simulink model "Plant_Model_W_Sensors_Un_biased"  (R2017b)
settings: Solver=VariableStepAuto  StartTime=0.0  StopTime=TF  FixedStep=0.001  MaxStep=1e-4  RelTol=1e-4
values from neighbouring files (symbols this model uses):
  Accel_bias = 1    [Model_W_MD_Sensors.m]
  Amps = C/1000    (= 0.7)    [Model_W_MD_Sensors.m]
  b = 1.144e-08    [Model_W_MD_Sensors.m]
  b_m = 2.415e-6    (= 2.415e-06)    [Model_W_MD_Sensors.m]
  CD = 0.7    [Model_W_MD_Sensors.m]
  d = 9.94e-10    [Model_W_MD_Sensors.m]
  g = 9.81    [Model_W_MD_Sensors.m]
  Grav_bias = g    (= 9.81)    [Model_W_MD_Sensors.m]
  Gyro_bias = .6    (= 0.6)    [Model_W_MD_Sensors.m]
  Ixx = 7.5*10^(-3)    (= 0.0075)    [Model_W_MD_Sensors.m]
  Iyy = 7.5*10^(-3)    (= 0.0075)    [Model_W_MD_Sensors.m]
  Izz = 1.3*10^(-2)    (= 0.013)    [Model_W_MD_Sensors.m]
  Jr = 6.5*10^(-7)    (= 6.5e-07)    [Model_W_MD_Sensors.m]
  Kemf = 0.00255    [Model_W_MD_Sensors.m]
  Kt = Kemf    (= 0.00255)    [Model_W_MD_Sensors.m]
  l = 0.23    [Model_W_MD_Sensors.m]
  L = 0.001*R    (= 0.000117)    [Model_W_MD_Sensors.m]
  m = weight/g    (= 0.0289500509684)    [Model_W_MD_Sensors.m]
  PD = 120    [Model_W_MD_Sensors.m]
  Phi_dot_bias = mean(Phi_dot)    [Model_W_MD_Sensors.m]
  Psi_dot_bias = mean(Psi_dot)    [Model_W_MD_Sensors.m]
  R = 0.117    [Model_W_MD_Sensors.m]
  Theta_dot_bias = mean(Theta_dot)    [Model_W_MD_Sensors.m]
  X_dot_dot_bias = mean(X_dot_dot)    [Model_W_MD_Sensors.m]
  Y_dot_dot_bias = mean(Y_dot_dot)    [Model_W_MD_Sensors.m]
  Z_dot_dot_bias = mean(Z_dot_dot)    [Model_W_MD_Sensors.m]
undefined symbols (not defined in the file or in its folder): Ion, Lithium
libraries: simulink x9, powerlib x2, electricdrivelib x1
settings Model: Creator=Nicky  LastModifiedBy=Nicky
settings SolverCC: ZeroCrossAlgorithm=Adaptive  AutoInsertRateTranBlk=on
settings DebuggingCC: MaxConsecutiveZCsMsg=none
settings CodeAppCC: StateflowObjectComments=on
settings SimscapeCC: SimscapeNormalizeSystem=off

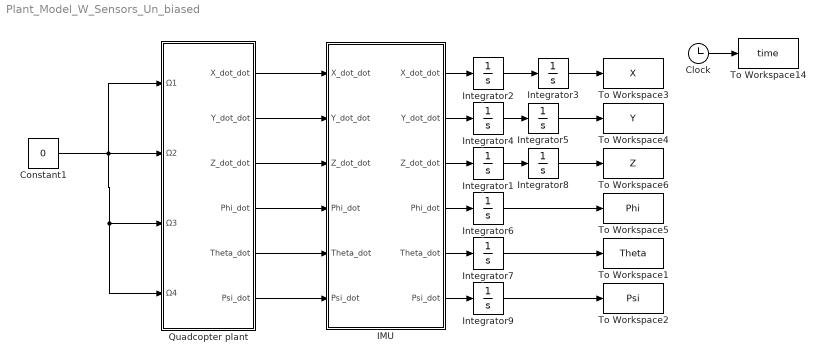
== system Plant_Model_W_Sensors_Un_biased ==
  Clock : Clock
  Constant1 : Constant  Value=0
  IMU : Subsystem
  Integrator{1..5,9} (6 alike) : Integrator
  Integrator6 : Integrator  WrapState=on
  Integrator7 : Integrator  WrapState=on
  Integrator8 : Integrator  LimitOutput=on  UpperSaturationLimit=0
  Quadcopter plant : Subsystem
  To Workspace1 : ToWorkspace  VariableName=Theta  SampleTime=0.001
      settings: Save2DSignal=2-D array (concatenate along first dimension)
  To Workspace14 : ToWorkspace  VariableName=time  SampleTime=0.001
      settings: Save2DSignal=2-D array (concatenate along first dimension)
  To Workspace2 : ToWorkspace  VariableName=Psi  SampleTime=0.001
      settings: Save2DSignal=2-D array (concatenate along first dimension)
  To Workspace3 : ToWorkspace  VariableName=X  SampleTime=0.001
      settings: Save2DSignal=2-D array (concatenate along first dimension)
  To Workspace4 : ToWorkspace  VariableName=Y  SampleTime=0.001
      settings: Save2DSignal=2-D array (concatenate along first dimension)
  To Workspace5 : ToWorkspace  VariableName=Phi  SampleTime=0.001
      settings: Save2DSignal=2-D array (concatenate along first dimension)
  To Workspace6 : ToWorkspace  VariableName=Z  SampleTime=0.001
      settings: Save2DSignal=2-D array (concatenate along first dimension)
  wires:
  Clock/1 -> To Workspace14/1
  Quadcopter plant/1(X_dot_dot) -> IMU/1(X_dot_dot)
  Quadcopter plant/2("Y_dot_dot ") -> IMU/2(Y_dot_dot)
  Quadcopter plant/3(Z_dot_dot) -> IMU/3(Z_dot_dot)
  Quadcopter plant/4(Phi_dot) -> IMU/4(Phi_dot)
  Quadcopter plant/5(Theta_dot) -> IMU/5(Theta_dot)
  Quadcopter plant/6(Psi_dot) -> IMU/6(Psi_dot)
  Constant1/1 -> Quadcopter plant/1(Ω1), Quadcopter plant/2(Ω2), Quadcopter plant/3(Ω3), Quadcopter plant/4(Ω4)
  Integrator4/1 -> Integrator5/1
  Integrator2/1 -> Integrator3/1
  Integrator3/1 -> To Workspace3/1
  IMU/1("X_dot_dot ") -> Integrator2/1
  IMU/2("Y_dot_dot ") -> Integrator4/1
  Integrator5/1 -> To Workspace4/1
  Integrator1/1 -> Integrator8/1
  IMU/3("Z_dot_dot ") -> Integrator1/1
  Integrator8/1 -> To Workspace6/1
  IMU/4("Phi_dot ") -> Integrator6/1
  Integrator6/1 -> To Workspace5/1
  IMU/5("Theta_dot ") -> Integrator7/1
  Integrator7/1 -> To Workspace1/1
  IMU/6("Psi_dot ") -> Integrator9/1
  Integrator9/1 -> To Workspace2/1

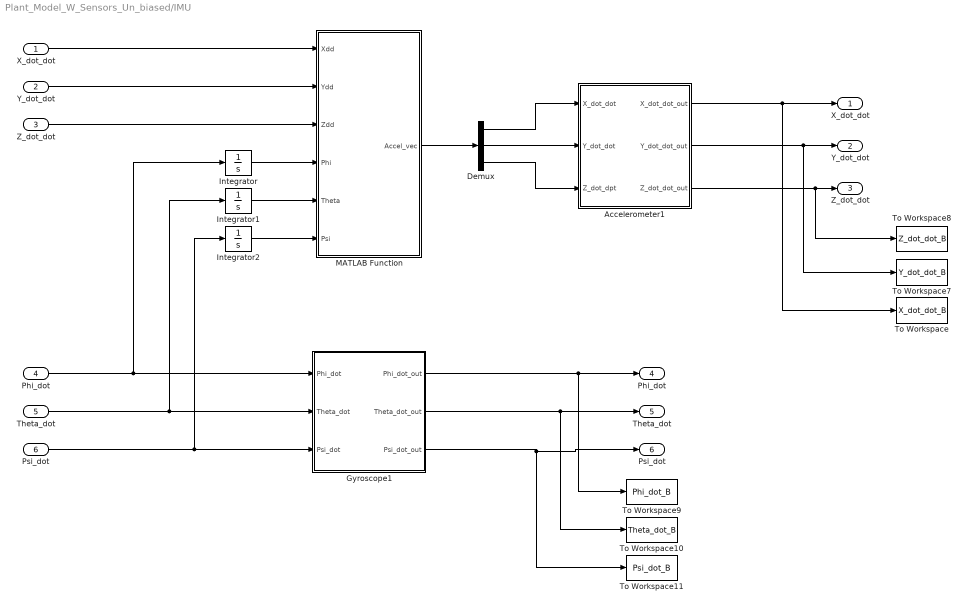
== system Plant_Model_W_Sensors_Un_biased/IMU ==
  X_dot_dot : Inport
  Y_dot_dot : Inport  Port=2
  Z_dot_dot : Inport  Port=3
  Phi_dot : Inport  Port=4
  Theta_dot : Inport  Port=5
  Psi_dot : Inport  Port=6
  Accelerometer1 : Subsystem
  Demux : Demux  Outputs=3
  Gyroscope1 : Subsystem
  Integrator : Integrator  WrapState=on
  Integrator1 : Integrator  WrapState=on
  Integrator2 : Integrator
  MATLAB Function : MATLAB Function  TreatAsAtomicUnit=on
  To Workspace : ToWorkspace  VariableName=X_dot_dot_B  SampleTime=0.001
      settings: Save2DSignal=2-D array (concatenate along first dimension)
  To Workspace10 : ToWorkspace  VariableName=Theta_dot_B  SampleTime=0.001
      settings: Save2DSignal=2-D array (concatenate along first dimension)
  To Workspace11 : ToWorkspace  VariableName=Psi_dot_B  SampleTime=0.001
      settings: Save2DSignal=2-D array (concatenate along first dimension)
  To Workspace7 : ToWorkspace  VariableName=Y_dot_dot_B  SampleTime=0.001
      settings: Save2DSignal=2-D array (concatenate along first dimension)
  To Workspace8 : ToWorkspace  VariableName=Z_dot_dot_B  SampleTime=0.001
      settings: Save2DSignal=2-D array (concatenate along first dimension)
  To Workspace9 : ToWorkspace  VariableName=Phi_dot_B  SampleTime=0.001
      settings: Save2DSignal=2-D array (concatenate along first dimension)
  "X_dot_dot " : Outport
  "Y_dot_dot " : Outport  Port=2
  "Z_dot_dot " : Outport  Port=3
  "Phi_dot " : Outport  Port=4
  "Theta_dot " : Outport  Port=5
  "Psi_dot " : Outport  Port=6
  wires:
  Phi_dot/1 -> Gyroscope1/1(Phi_dot), Integrator/1
  Theta_dot/1 -> Gyroscope1/2(Theta_dot), Integrator1/1
  Psi_dot/1 -> Gyroscope1/3(Psi_dot), Integrator2/1
  X_dot_dot/1 -> MATLAB Function/1(Xdd)
  Y_dot_dot/1 -> MATLAB Function/2(Ydd)
  Z_dot_dot/1 -> MATLAB Function/3(Zdd)
  Integrator/1 -> MATLAB Function/4(Phi)
  Integrator2/1 -> MATLAB Function/6(Psi)
  Integrator1/1 -> MATLAB Function/5(Theta)
  MATLAB Function/1(Accel_vec) -> Demux/1
  Demux/2 -> Accelerometer1/2("Y_dot_dot ")
  Demux/1 -> Accelerometer1/1(X_dot_dot)
  Demux/3 -> Accelerometer1/3("Z_dot_dpt ")
  Accelerometer1/2(Y_dot_dot_out) -> To Workspace7/1, "Y_dot_dot "/1
  Accelerometer1/3(Z_dot_dot_out) -> "Z_dot_dot "/1, To Workspace8/1
  Accelerometer1/1(X_dot_dot_out) -> "X_dot_dot "/1, To Workspace/1
  Gyroscope1/2(Theta_dot_out) -> "Theta_dot "/1, To Workspace10/1
  Gyroscope1/1(Phi_dot_out) -> "Phi_dot "/1, To Workspace9/1
  Gyroscope1/3(Psi_dot_out) -> "Psi_dot "/1, To Workspace11/1

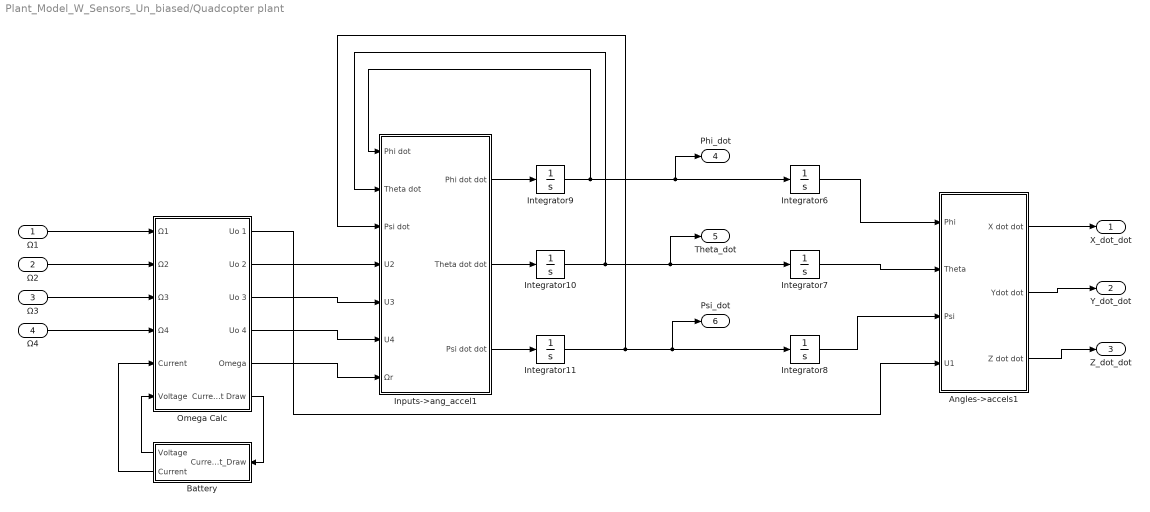
== system Plant_Model_W_Sensors_Un_biased/Quadcopter plant ==
  Ω1 : Inport
  Ω2 : Inport  Port=2
  Ω3 : Inport  Port=3
  Ω4 : Inport  Port=4
  Angles->accels1 : Subsystem
  Battery : Subsystem
  Inputs->ang_accel1 : Subsystem
  Integrator10 : Integrator  IgnoreLimit=on
  Integrator11 : Integrator  UpperSaturationLimit=10000  LowerSaturationLimit=-10000
  Integrator6 : Integrator  WrapState=on
  Integrator7 : Integrator  WrapState=on
  Integrator8 : Integrator
  Integrator9 : Integrator
  Omega Calc : Subsystem
  X_dot_dot : Outport
  "Y_dot_dot " : Outport  Port=2
  Z_dot_dot : Outport  Port=3
  Phi_dot : Outport  Port=4
  Theta_dot : Outport  Port=5
  Psi_dot : Outport  Port=6
  wires:
  Integrator8/1 -> Angles->accels1/3(Psi)
  Integrator7/1 -> Angles->accels1/2(Theta)
  Integrator6/1 -> Angles->accels1/1(Phi)
  Inputs->ang_accel1/2(Theta dot dot) -> Integrator10/1
  Inputs->ang_accel1/1(Phi dot dot) -> Integrator9/1
  Inputs->ang_accel1/3(Psi dot dot) -> Integrator11/1
  Omega Calc/5(Omega) -> Inputs->ang_accel1/7(Ωr)
  Omega Calc/4(Uo 4) -> Inputs->ang_accel1/6(U4)
  Omega Calc/3(Uo 3) -> Inputs->ang_accel1/5(U3)
  Omega Calc/2(Uo 2) -> Inputs->ang_accel1/4(U2)
  Omega Calc/1(Uo 1) -> Angles->accels1/4(U1)
  Ω1/1 -> Omega Calc/1(Ω1)
  Ω2/1 -> Omega Calc/2(Ω2)
  Ω3/1 -> Omega Calc/3(Ω3)
  Ω4/1 -> Omega Calc/4(Ω4)
  Integrator9/1 -> Inputs->ang_accel1/1(Phi dot), Phi_dot/1, Integrator6/1
  Integrator11/1 -> Inputs->ang_accel1/3(Psi dot), Integrator8/1, Psi_dot/1
  Integrator10/1 -> Inputs->ang_accel1/2(Theta dot), Integrator7/1, Theta_dot/1
  Angles->accels1/1(X dot dot) -> X_dot_dot/1
  Angles->accels1/2(Ydot dot) -> "Y_dot_dot "/1
  Angles->accels1/3(Z dot dot) -> Z_dot_dot/1
  Omega Calc/6(Current Draw) -> Battery/1(Current_Draw)
  Battery/1(Voltage) -> Omega Calc/6(Voltage)
  Battery/2(Current) -> Omega Calc/5(Current)

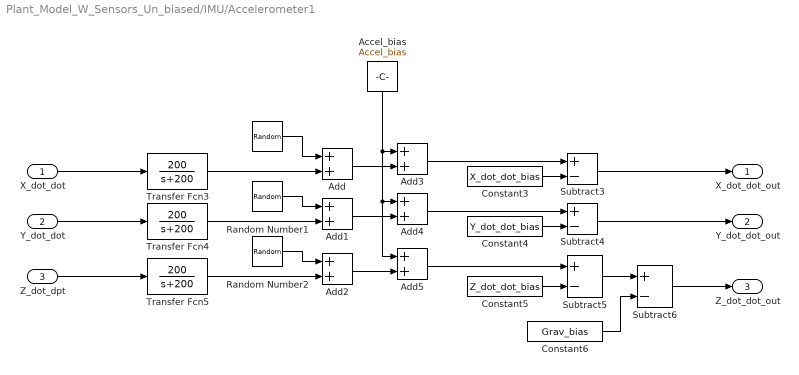
== system Plant_Model_W_Sensors_Un_biased/IMU/Accelerometer1 ==
  X_dot_dot : Inport
  "Y_dot_dot " : Inport  Port=2
  "Z_dot_dpt " : Inport  Port=3
  " " : RandomNumber  Variance=0.0001  Seed=1  SampleTime=0.001
  Accel_bias : Constant  Value=Accel_bias
  Add{,1..5} (6 alike) : Sum
  Constant3 : Constant  Value=X_dot_dot_bias
  Constant4 : Constant  Value=Y_dot_dot_bias
  Constant5 : Constant  Value=Z_dot_dot_bias
  Constant6 : Constant  Value=Grav_bias
  Random Number1 : RandomNumber  Variance=0.0001  Seed=2  SampleTime=0.001
  Random Number2 : RandomNumber  Mean=0.000  Variance=0.0001  Seed=3  SampleTime=0.001
  Subtract{3..6} (4 alike) : Sum  Inputs=+-
  Transfer Fcn3 : TransferFcn  Numerator=[200]  Denominator=[1 200]
  Transfer Fcn4 : TransferFcn  Numerator=[200]  Denominator=[1 200]
  Transfer Fcn5 : TransferFcn  Numerator=[200]  Denominator=[1 200]
  X_dot_dot_out : Outport
  Y_dot_dot_out : Outport  Port=2
  Z_dot_dot_out : Outport  Port=3
  wires:
  Constant6/1 -> Subtract6/2
  Constant4/1 -> Subtract4/2
  Constant3/1 -> Subtract3/2
  Constant5/1 -> Subtract5/2
  Subtract5/1 -> Subtract6/1
  X_dot_dot/1 -> Transfer Fcn3/1
  "Y_dot_dot "/1 -> Transfer Fcn4/1
  Accel_bias/1 -> Add5/1, Add4/1, Add3/1
  Add/1 -> Add3/2
  Add2/1 -> Add5/2
  Add1/1 -> Add4/2
  Add3/1 -> Subtract3/1
  Add4/1 -> Subtract4/1
  Add5/1 -> Subtract5/1
  " "/1 -> Add/1
  Random Number1/1 -> Add1/1
  Random Number2/1 -> Add2/1
  "Z_dot_dpt "/1 -> Transfer Fcn5/1
  Subtract3/1 -> X_dot_dot_out/1
  Subtract4/1 -> Y_dot_dot_out/1
  Subtract6/1 -> Z_dot_dot_out/1
  Transfer Fcn3/1 -> Add/2
  Transfer Fcn5/1 -> Add2/2
  Transfer Fcn4/1 -> Add1/2

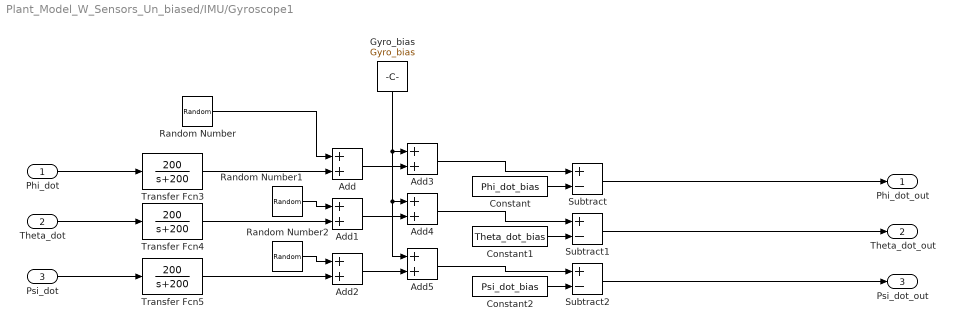
== system Plant_Model_W_Sensors_Un_biased/IMU/Gyroscope1 ==
  Phi_dot : Inport
  Theta_dot : Inport  Port=2
  Psi_dot : Inport  Port=3
  Add{,1..5} (6 alike) : Sum
  Constant : Constant  Value=Phi_dot_bias
  Constant1 : Constant  Value=Theta_dot_bias
  Constant2 : Constant  Value=Psi_dot_bias
  Gyro_bias : Constant  Value=Gyro_bias
  Random Number : RandomNumber  Variance=0.0001  Seed=4  SampleTime=0.001
  Random Number1 : RandomNumber  Variance=0.0001  Seed=5  SampleTime=0.001
  Random Number2 : RandomNumber  Variance=0.0001  Seed=6  SampleTime=0.001
  Subtract : Sum  Inputs=+-
  Subtract1 : Sum  Inputs=+-
  Subtract2 : Sum  Inputs=+-
  Transfer Fcn3 : TransferFcn  Numerator=[200]  Denominator=[1 200]
  Transfer Fcn4 : TransferFcn  Numerator=[200]  Denominator=[1 200]
  Transfer Fcn5 : TransferFcn  Numerator=[200]  Denominator=[1 200]
  Phi_dot_out : Outport
  Theta_dot_out : Outport  Port=2
  Psi_dot_out : Outport  Port=3
  wires:
  Constant/1 -> Subtract/2
  Constant2/1 -> Subtract2/2
  Constant1/1 -> Subtract1/2
  Phi_dot/1 -> Transfer Fcn3/1
  Theta_dot/1 -> Transfer Fcn4/1
  Psi_dot/1 -> Transfer Fcn5/1
  Add/1 -> Add3/2
  Add1/1 -> Add4/2
  Add2/1 -> Add5/2
  Add5/1 -> Subtract2/1
  Add3/1 -> Subtract/1
  Add4/1 -> Subtract1/1
  Gyro_bias/1 -> Add5/1, Add4/1, Add3/1
  Random Number/1 -> Add/1
  Random Number1/1 -> Add1/1
  Random Number2/1 -> Add2/1
  Subtract/1 -> Phi_dot_out/1
  Subtract1/1 -> Theta_dot_out/1
  Subtract2/1 -> Psi_dot_out/1
  Transfer Fcn3/1 -> Add/2
  Transfer Fcn5/1 -> Add2/2
  Transfer Fcn4/1 -> Add1/2

== system Plant_Model_W_Sensors_Un_biased/Quadcopter plant/Angles->accels1 ==
  Phi : Inport
  Theta : Inport  Port=2
  Psi : Inport  Port=3
  U1 : Inport  Port=4
  Constant : Constant  Value=m
  Divide : Product  Inputs=*/
  Subsystem : Subsystem
  Subsystem1 : Subsystem
  Subsystem2 : Subsystem
  X dot dot : Outport
  Ydot dot : Outport  Port=2
  Z dot dot : Outport  Port=3
  wires:
  Phi/1 -> Subsystem1/1(Phi), Subsystem2/1(Phi), Subsystem/1(Phi)
  U1/1 -> Divide/1
  Constant/1 -> Divide/2
  Divide/1 -> Subsystem2/3(U1/m), Subsystem1/4(U1/M), Subsystem/4(U1/M)
  Subsystem/1(X_dot_dot) -> X dot dot/1
  Subsystem1/1(Y_dot_dot) -> Ydot dot/1
  Subsystem2/1(Z_dot_dot) -> Z dot dot/1
  Theta/1 -> Subsystem2/2(Theta), Subsystem1/2(Theta), Subsystem/2(Theta)
  Psi/1 -> Subsystem/3(Psi), Subsystem1/3(Psi)

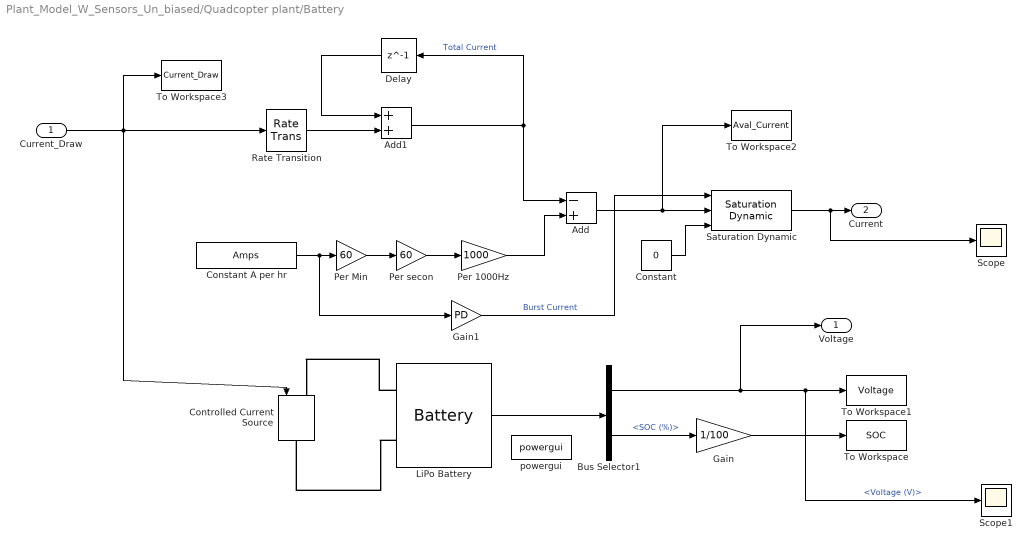
== system Plant_Model_W_Sensors_Un_biased/Quadcopter plant/Battery ==
  Current_Draw : Inport
  Add : Sum  Inputs=-+
  Add1 : Sum
  Bus Selector1 : BusSelector  OutputSignals=Voltage (V),SOC (%)
  Constant : Constant  Value=0
  Constant A per hr : Constant  Value=Amps
  Controlled Current Source : powerlib/Electrical Sources/Controlled Current Source  Initialize=on  Source_Type=DC  Amplitude=0  Phase=0  Frequency=0  Measurements=None
  Delay : Delay  DelayLength=1  InitialCondition=0
  Gain : Gain  Gain=1/100
  Gain1 : Gain  Gain=PD
  "LiPo Battery " : electricdrivelib/Extra Sources/Battery  BatType=Lithium-Ion  ShowTempParam=off  ThermalPreset=no  ShowAgeParam=off  NomV=11.1  NomQ=.7  SOC=100  Batt_Tr=1  PresetModel=off  MaxQ=0.7  MinV=8.325  FullV=11.75  Dis_rate=.7  R=.08  Normal_OP=.7  expZone="[11.75   0.5]"  current=CD*Amps  Units=Ampere-hour  Tci=20  NomT=25  T2=0  MaxQ2=2.208  FullV2=3.45  Normal_OP2=2.8  expZone2="[3.22        0.23]"  Rca=0.6  ti=1000  Dp=0  Neq0=0  Tsim=1e6  Ta1=25  Qeol=5.4*0.9  Reol=0.013333*1.2  Char_age=[2.3478, 3]  Dis_age=[2.3478, 10]  N1=1500  N2=10500  N3=1000  N4=1400  Ta2=45  N5=950
  Per 1000Hz : Gain  Gain=1000
  Per Min : Gain  Gain=60
  Per secon : Gain  Gain=60
  Rate Transition : RateTransition  OutPortSampleTimeMultiple=0  OutPortSampleTime=0.001
  Saturation Dynamic : simulink/Discontinuities/Saturation Dynamic  OutMin=[]  OutMax=[]  OutDataTypeStr=Inherit: Same as second input  OutDataType=fixdt(1, 16)  OutScaling=2^-10  DoSatur=off
  Scope : Scope
  Scope1 : Scope
  To Workspace : ToWorkspace  VariableName=SOC  SampleTime=.1
      settings: Save2DSignal=2-D array (concatenate along first dimension)
  To Workspace1 : ToWorkspace  VariableName=Voltage  SampleTime=.1
      settings: Save2DSignal=2-D array (concatenate along first dimension)
  To Workspace2 : ToWorkspace  VariableName=Aval_Current  SampleTime=.1
      settings: Save2DSignal=2-D array (concatenate along first dimension)
  To Workspace3 : ToWorkspace  VariableName=Current_Draw  SampleTime=.1
      settings: Save2DSignal=2-D array (concatenate along first dimension)
  powergui : powerlib/powergui  SimulationMode=Continuous  SampleTime=0.001  frequency=60  Iterations=50  frequencyindice=0  Pbase=100e6  ErrMax=1e-4  UnitsV=kV  UnitsW=MW  buscounter=0  FunctionMessages=off  echomessages=off  EnableUseOfTLC=off  CurrentSourceSwitches=off  DisableSnubberDevices=off  DisableRonSwitches=off  DisableVfSwitches=off  DisplayEquations=off  SolverType=Tustin/Backward Euler (TBE)  Interpol=off  ExternalGateDelay=off  methode=off  Ts=100  x0status=blocks  SPID=on  SwTol=0  HookPort=off  RestoreLinks=warning  ResistiveCurrentMeasurement=off  Frange=[0:2:500]  Ylog=off  Xlog=on  ShowGrid=off  save=off  variable=ZData  structure=0  ZoomFFT=on  StartTime=0.0  cycles=1  DisplayStyle=1  fundamental=60  FreqAxis=off  MaxFrequency=1000  frequencyindicesteady=1  RmsSteady=1  display=off
  Voltage : Outport
  Current : Outport  Port=2
  wires:
  Per Min/1 -> Per secon/1
  Constant A per hr/1 -> Gain1/1, Per Min/1
  Per secon/1 -> Per 1000Hz/1
  Per 1000Hz/1 -> Add/2
  Add1/1 -> Add/1, Delay/1  "Total Current"
  Rate Transition/1 -> Add1/2
  Delay/1 -> Add1/1
  Constant/1 -> Saturation Dynamic/3
  Current_Draw/1 -> To Workspace3/1, Controlled Current Source/1, Rate Transition/1
  Bus Selector1/1 -> Voltage/1, Scope1/1, To Workspace1/1  "<Voltage (V)>"
  Bus Selector1/2 -> Gain/1  "<SOC (%)>"
  Gain/1 -> To Workspace/1
  "LiPo Battery "/1 -> Bus Selector1/1
  Add/1 -> To Workspace2/1, Saturation Dynamic/2
  Saturation Dynamic/1 -> Scope/1, Current/1
  Gain1/1 -> Saturation Dynamic/1  "Burst Current"
  connections:
  "LiPo Battery "/LConn1 -- Controlled Current Source/LConn1
  "LiPo Battery "/LConn2 -- Controlled Current Source/RConn1

== system Plant_Model_W_Sensors_Un_biased/Quadcopter plant/Inputs->ang_accel1 ==
  Phi dot : Inport
  Theta dot : Inport  Port=2
  Psi dot : Inport  Port=3
  U2 : Inport  Port=4
  U3 : Inport  Port=5
  U4 : Inport  Port=6
  Ωr : Inport  Port=7
  Subsystem : Subsystem
  Subsystem1 : Subsystem
  Subsystem2 : Subsystem
  Phi dot dot : Outport
  Theta dot dot : Outport  Port=2
  Psi dot dot : Outport  Port=3
  wires:
  U3/1 -> Subsystem2/3(U3)
  U4/1 -> Subsystem1/3(U4)
  Subsystem/1(Phi_dot_dot) -> Phi dot dot/1
  U2/1 -> Subsystem/1(U2)
  Ωr/1 -> Subsystem/4(Ωr), Subsystem2/1(Ωr)
  Psi dot/1 -> Subsystem2/2(Psi_dot), Subsystem/3(Psi_dot)
  Subsystem2/1(Theta_dot_dot) -> Theta dot dot/1
  Subsystem1/1(Psi_dot_dot) -> Psi dot dot/1
  Theta dot/1 -> Subsystem/2(Theta_dot), Subsystem1/2(Theta_dot)
  Phi dot/1 -> Subsystem2/4(Phi_dot), Subsystem1/1(Phi_dot)

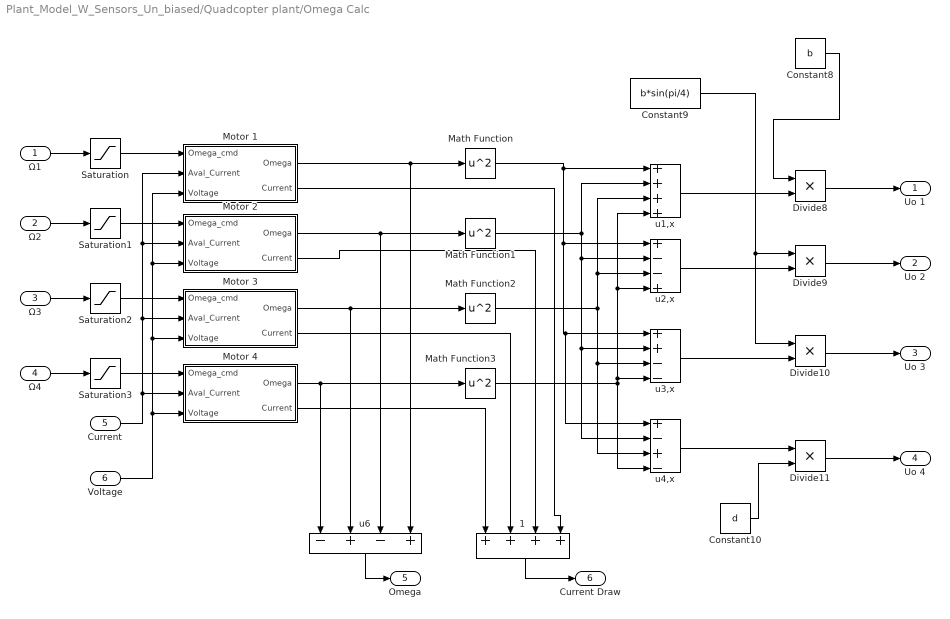
== system Plant_Model_W_Sensors_Un_biased/Quadcopter plant/Omega Calc ==
  Ω1 : Inport
  Ω2 : Inport  Port=2
  Ω3 : Inport  Port=3
  Ω4 : Inport  Port=4
  Current : Inport  Port=5
  Voltage : Inport  Port=6
  " 1" : Sum  Inputs=++++
  " Motor 1" : Subsystem
  " Motor 2" : Subsystem
  " Motor 3" : Subsystem
  " Motor 4" : Subsystem
  Constant10 : Constant  Value=d
  Constant8 : Constant  Value=b
  Constant9 : Constant  Value=b*sin(pi/4)
  Divide{8..11} (4 alike) : Product  Inputs=**
  Math Function{,1..3} (4 alike) : Math  Operator=square  SaturateOnIntegerOverflow=on
  Saturation{,1..3} (4 alike) : Saturate  UpperLimit=inf  LowerLimit=0
  u1,x : Sum  Inputs=++++
  u2,x : Sum  Inputs=+--+
  u3,x : Sum  Inputs=++--
  u4,x : Sum  Inputs=+-+-
  u6 : Sum  Inputs=-+-+
  Uo 1 : Outport
  Uo 2 : Outport  Port=2
  Uo 3 : Outport  Port=3
  Uo 4 : Outport  Port=4
  Omega : Outport  Port=5
  Current Draw : Outport  Port=6
  wires:
  Constant10/1 -> Divide11/2
  u4,x/1 -> Divide11/1
  u3,x/1 -> Divide10/2
  u2,x/1 -> Divide9/2
  Constant9/1 -> Divide10/1, Divide9/1
  u1,x/1 -> Divide8/2
  Constant8/1 -> Divide8/1
  u6/1 -> Omega/1
  Divide8/1 -> Uo 1/1
  Divide9/1 -> Uo 2/1
  Divide10/1 -> Uo 3/1
  Divide11/1 -> Uo 4/1
  " Motor 1"/1(Omega) -> u6/4, Math Function/1
  " Motor 2"/1(Omega) -> u6/3, Math Function1/1
  " Motor 3"/1(Omega) -> u6/2, Math Function2/1
  " Motor 4"/1(Omega) -> u6/1, Math Function3/1
  " 1"/1 -> Current Draw/1
  Ω1/1 -> Saturation/1
  Ω2/1 -> Saturation1/1
  Ω3/1 -> Saturation2/1
  Ω4/1 -> Saturation3/1
  Saturation/1 -> " Motor 1"/1(Omega_cmd)
  Saturation1/1 -> " Motor 2"/1(Omega_cmd)
  Saturation2/1 -> " Motor 3"/1(Omega_cmd)
  Saturation3/1 -> " Motor 4"/1(Omega_cmd)
  Current/1 -> " Motor 4"/2(Aval_Current), " Motor 3"/2(Aval_Current), " Motor 2"/2(Aval_Current), " Motor 1"/2(Aval_Current)
  Voltage/1 -> " Motor 4"/3(Voltage), " Motor 3"/3(Voltage), " Motor 2"/3(Voltage), " Motor 1"/3(Voltage)
  " Motor 4"/2("Current ") -> " 1"/1
  " Motor 3"/2("Current ") -> " 1"/2
  " Motor 2"/2("Current ") -> " 1"/3
  " Motor 1"/2("Current ") -> " 1"/4
  Math Function/1 -> u4,x/1, u3,x/1, u2,x/1, u1,x/1
  Math Function1/1 -> u4,x/2, u3,x/2, u2,x/2, u1,x/2
  Math Function2/1 -> u4,x/3, u3,x/3, u1,x/3, u2,x/3
  Math Function3/1 -> u4,x/4, u1,x/4, u2,x/4, u3,x/4

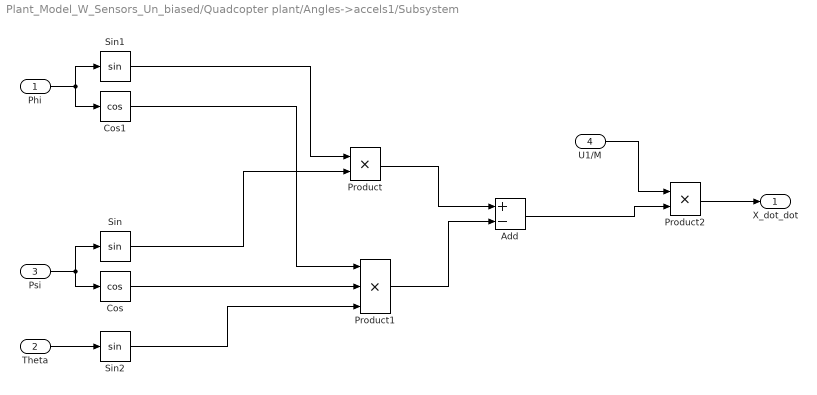
== system Plant_Model_W_Sensors_Un_biased/Quadcopter plant/Angles->accels1/Subsystem ==
  Phi : Inport
  Theta : Inport  Port=2
  Psi : Inport  Port=3
  U1/M : Inport  Port=4
  Add : Sum  Inputs=+-
  Cos : Trigonometry  Operator=cos
  Cos1 : Trigonometry  Operator=cos
  Product : Product
  Product1 : Product  Inputs=3
  Product2 : Product
  Sin : Trigonometry
  Sin1 : Trigonometry
  Sin2 : Trigonometry
  X_dot_dot : Outport
  wires:
  Product2/1 -> X_dot_dot/1
  Product1/1 -> Add/2
  Product/1 -> Add/1
  U1/M/1 -> Product2/1
  Add/1 -> Product2/2
  Psi/1 -> Cos/1, Sin/1
  Phi/1 -> Cos1/1, Sin1/1
  Theta/1 -> Sin2/1
  Cos1/1 -> Product1/1
  Cos/1 -> Product1/2
  Sin2/1 -> Product1/3
  Sin1/1 -> Product/1
  Sin/1 -> Product/2

== system Plant_Model_W_Sensors_Un_biased/Quadcopter plant/Angles->accels1/Subsystem1 ==
  Phi : Inport
  Theta : Inport  Port=2
  Psi : Inport  Port=3
  U1/M : Inport  Port=4
  Add1 : Sum
  Cos : Trigonometry  Operator=cos
  Cos1 : Trigonometry  Operator=cos
  Product3 : Product
  Product4 : Product  Inputs=3
  Product5 : Product
  Sin : Trigonometry
  Sin1 : Trigonometry
  Sin2 : Trigonometry
  Y_dot_dot : Outport
  wires:
  Psi/1 -> Sin/1, Cos/1
  Phi/1 -> Cos1/1, Sin1/1
  Theta/1 -> Sin2/1
  Product5/1 -> Y_dot_dot/1
  Add1/1 -> Product5/2
  Product4/1 -> Add1/2
  U1/M/1 -> Product5/1
  Product3/1 -> Add1/1
  Cos1/1 -> Product4/1
  Sin/1 -> Product4/2
  Sin2/1 -> Product4/3
  Sin1/1 -> Product3/1
  Cos/1 -> Product3/2

== system Plant_Model_W_Sensors_Un_biased/Quadcopter plant/Angles->accels1/Subsystem2 ==
  Phi : Inport
  Theta : Inport  Port=2
  U1/m : Inport  Port=3
  Add2 : Sum  Inputs=+-
  Constant2 : Constant  Value=g
  Cos : Trigonometry  Operator=cos
  Cos1 : Trigonometry  Operator=cos
  Product6 : Product  Inputs=3
  Z_dot_dot : Outport
  wires:
  Phi/1 -> Cos1/1
  Theta/1 -> Cos/1
  U1/m/1 -> Product6/3
  Constant2/1 -> Add2/1
  Cos/1 -> Product6/1
  Product6/1 -> Add2/2
  Cos1/1 -> Product6/2
  Add2/1 -> Z_dot_dot/1

== system Plant_Model_W_Sensors_Un_biased/Quadcopter plant/Inputs->ang_accel1/Subsystem ==
  U2 : Inport
  Theta_dot : Inport  Port=2
  Psi_dot : Inport  Port=3
  Ωr : Inport  Port=4
  Add : Sum  Inputs=+++
  Constant : Constant  Value=Iyy-Izz
  Constant1 : Constant  Value=Jr
  Constant2 : Constant  Value=l
  Constant3 : Constant  Value=Ixx
  Divide : Product  Inputs=*/
  Product : Product  Inputs=3
  Product1 : Product  Inputs=3
  Product2 : Product
  Phi_dot_dot : Outport
  wires:
  Psi_dot/1 -> Product/2
  Theta_dot/1 -> Product/1, Product1/3
  Constant/1 -> Product/3
  Ωr/1 -> Product1/2
  Constant1/1 -> Product1/1
  U2/1 -> Product2/2
  Constant2/1 -> Product2/1
  Product1/1 -> Add/2
  Product2/1 -> Add/1
  Product/1 -> Add/3
  Add/1 -> Divide/1
  Constant3/1 -> Divide/2
  Divide/1 -> Phi_dot_dot/1

== system Plant_Model_W_Sensors_Un_biased/Quadcopter plant/Inputs->ang_accel1/Subsystem1 ==
  Phi_dot : Inport
  Theta_dot : Inport  Port=2
  U4 : Inport  Port=3
  Add2 : Sum
  Constant11 : Constant  Value=Izz
  Constant8 : Constant  Value=Ixx-Iyy
  Divide2 : Product  Inputs=*/
  Product6 : Product  Inputs=3
  Psi_dot_dot : Outport
  wires:
  Theta_dot/1 -> Product6/1
  Phi_dot/1 -> Product6/2
  Constant8/1 -> Product6/3
  Add2/1 -> Divide2/1
  Constant11/1 -> Divide2/2
  Divide2/1 -> Psi_dot_dot/1
  Product6/1 -> Add2/2
  U4/1 -> Add2/1

== system Plant_Model_W_Sensors_Un_biased/Quadcopter plant/Inputs->ang_accel1/Subsystem2 ==
  Ωr : Inport
  Psi_dot : Inport  Port=2
  U3 : Inport  Port=3
  Phi_dot : Inport  Port=4
  Add1 : Sum  Inputs=+-+
  Constant4 : Constant  Value=Izz-Ixx
  Constant5 : Constant  Value=Jr
  Constant6 : Constant  Value=l
  Constant7 : Constant  Value=Iyy
  Divide1 : Product  Inputs=*/
  Product3 : Product  Inputs=3
  Product4 : Product  Inputs=3
  Product5 : Product
  Theta_dot_dot : Outport
  wires:
  Psi_dot/1 -> Product3/2
  Phi_dot/1 -> Product3/1, Product4/3
  Ωr/1 -> Product4/2
  Constant4/1 -> Product3/3
  Constant5/1 -> Product4/1
  U3/1 -> Product5/2
  Constant6/1 -> Product5/1
  Product4/1 -> Add1/2
  Product5/1 -> Add1/1
  Product3/1 -> Add1/3
  Add1/1 -> Divide1/1
  Constant7/1 -> Divide1/2
  Divide1/1 -> Theta_dot_dot/1

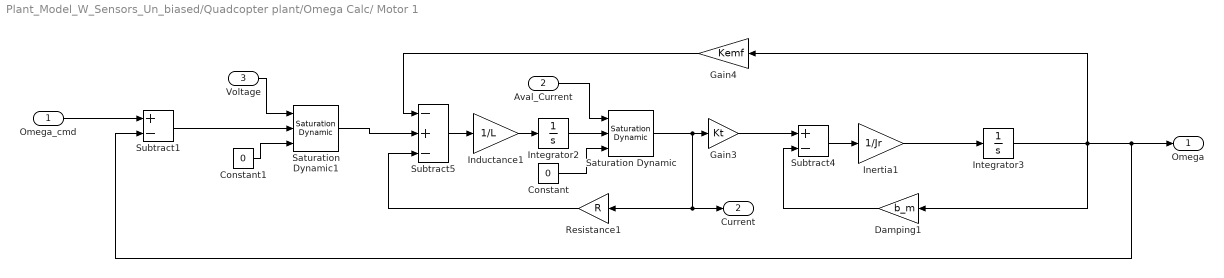
== system Plant_Model_W_Sensors_Un_biased/Quadcopter plant/Omega Calc/ Motor 1 ==
  Omega_cmd : Inport
  Aval_Current : Inport  Port=2
  Voltage : Inport  Port=3
  Constant : Constant  Value=0
  Constant1 : Constant  Value=0
  Damping1 : Gain  Gain=b_m
  Gain3 : Gain  Gain=Kt
  Gain4 : Gain  Gain=Kemf
  Inductance1 : Gain  Gain=1/L
  Inertia1 : Gain  Gain=1/Jr
  Integrator2 : Integrator  LimitOutput=on  LowerSaturationLimit=0
  Integrator3 : Integrator  LimitOutput=on  LowerSaturationLimit=0
  Resistance1 : Gain  Gain=R
  Saturation Dynamic : simulink/Discontinuities/Saturation Dynamic  OutMin=[]  OutMax=[]  OutDataTypeStr=Inherit: Same as second input  OutDataType=fixdt(1, 16)  OutScaling=2^-10  DoSatur=off
  Saturation Dynamic1 : simulink/Discontinuities/Saturation Dynamic  OutMin=[]  OutMax=[]  OutDataTypeStr=Inherit: Same as second input  OutDataType=fixdt(1, 16)  OutScaling=2^-10  DoSatur=off
  Subtract1 : Sum  Inputs=+-
  Subtract4 : Sum  Inputs=+-
  Subtract5 : Sum  Inputs=-+-
  Omega : Outport
  "Current " : Outport  Port=2
  wires:
  Inductance1/1 -> Integrator2/1
  Inertia1/1 -> Integrator3/1
  Resistance1/1 -> Subtract5/3
  Damping1/1 -> Subtract4/2
  Subtract5/1 -> Inductance1/1
  Saturation Dynamic1/1 -> Subtract5/2
  Gain4/1 -> Subtract5/1
  Subtract4/1 -> Inertia1/1
  Gain3/1 -> Subtract4/1
  Omega_cmd/1 -> Subtract1/1
  Integrator3/1 -> Subtract1/2, Omega/1, Damping1/1, Gain4/1
  Constant/1 -> Saturation Dynamic/3
  Aval_Current/1 -> Saturation Dynamic/1
  Integrator2/1 -> Saturation Dynamic/2
  Voltage/1 -> Saturation Dynamic1/1
  Constant1/1 -> Saturation Dynamic1/3
  Subtract1/1 -> Saturation Dynamic1/2
  Saturation Dynamic/1 -> Resistance1/1, "Current "/1, Gain3/1

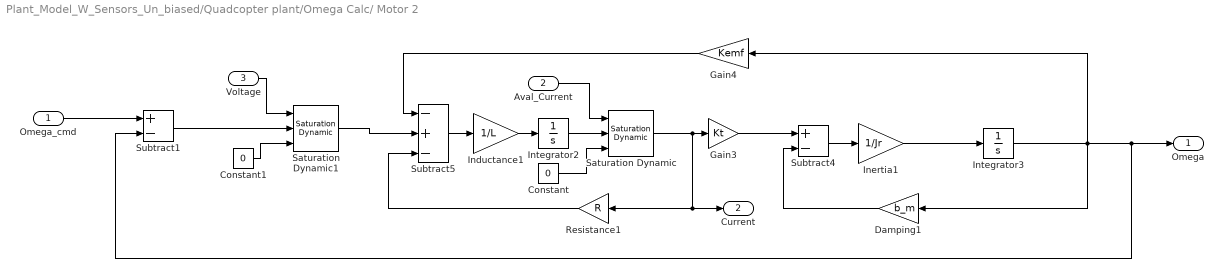
== system Plant_Model_W_Sensors_Un_biased/Quadcopter plant/Omega Calc/ Motor 2 ==
  Omega_cmd : Inport
  Aval_Current : Inport  Port=2
  Voltage : Inport  Port=3
  Constant : Constant  Value=0
  Constant1 : Constant  Value=0
  Damping1 : Gain  Gain=b_m
  Gain3 : Gain  Gain=Kt
  Gain4 : Gain  Gain=Kemf
  Inductance1 : Gain  Gain=1/L
  Inertia1 : Gain  Gain=1/Jr
  Integrator2 : Integrator  LimitOutput=on  LowerSaturationLimit=0
  Integrator3 : Integrator  LimitOutput=on  LowerSaturationLimit=0
  Resistance1 : Gain  Gain=R
  Saturation Dynamic : simulink/Discontinuities/Saturation Dynamic  OutMin=[]  OutMax=[]  OutDataTypeStr=Inherit: Same as second input  OutDataType=fixdt(1, 16)  OutScaling=2^-10  DoSatur=off
  Saturation Dynamic1 : simulink/Discontinuities/Saturation Dynamic  OutMin=[]  OutMax=[]  OutDataTypeStr=Inherit: Same as second input  OutDataType=fixdt(1, 16)  OutScaling=2^-10  DoSatur=off
  Subtract1 : Sum  Inputs=+-
  Subtract4 : Sum  Inputs=+-
  Subtract5 : Sum  Inputs=-+-
  Omega : Outport
  "Current " : Outport  Port=2
  wires:
  Inductance1/1 -> Integrator2/1
  Inertia1/1 -> Integrator3/1
  Resistance1/1 -> Subtract5/3
  Damping1/1 -> Subtract4/2
  Subtract5/1 -> Inductance1/1
  Saturation Dynamic1/1 -> Subtract5/2
  Gain4/1 -> Subtract5/1
  Subtract4/1 -> Inertia1/1
  Gain3/1 -> Subtract4/1
  Omega_cmd/1 -> Subtract1/1
  Integrator3/1 -> Subtract1/2, Omega/1, Damping1/1, Gain4/1
  Constant/1 -> Saturation Dynamic/3
  Aval_Current/1 -> Saturation Dynamic/1
  Integrator2/1 -> Saturation Dynamic/2
  Voltage/1 -> Saturation Dynamic1/1
  Constant1/1 -> Saturation Dynamic1/3
  Subtract1/1 -> Saturation Dynamic1/2
  Saturation Dynamic/1 -> Resistance1/1, "Current "/1, Gain3/1

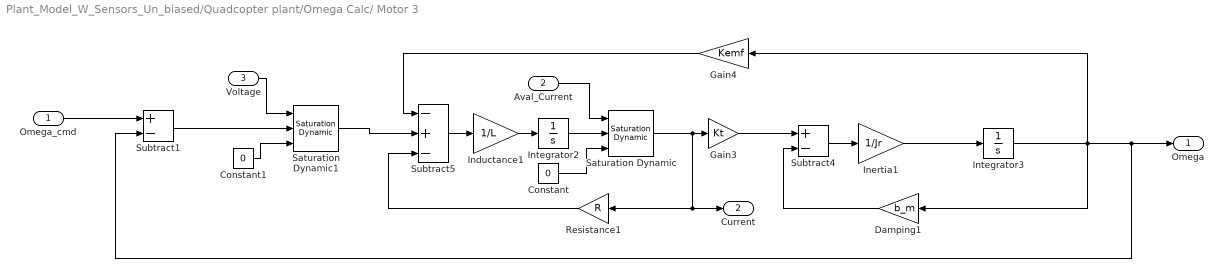
== system Plant_Model_W_Sensors_Un_biased/Quadcopter plant/Omega Calc/ Motor 3 ==
  Omega_cmd : Inport
  Aval_Current : Inport  Port=2
  Voltage : Inport  Port=3
  Constant : Constant  Value=0
  Constant1 : Constant  Value=0
  Damping1 : Gain  Gain=b_m
  Gain3 : Gain  Gain=Kt
  Gain4 : Gain  Gain=Kemf
  Inductance1 : Gain  Gain=1/L
  Inertia1 : Gain  Gain=1/Jr
  Integrator2 : Integrator  LimitOutput=on  LowerSaturationLimit=0
  Integrator3 : Integrator  LimitOutput=on  LowerSaturationLimit=0
  Resistance1 : Gain  Gain=R
  Saturation Dynamic : simulink/Discontinuities/Saturation Dynamic  OutMin=[]  OutMax=[]  OutDataTypeStr=Inherit: Same as second input  OutDataType=fixdt(1, 16)  OutScaling=2^-10  DoSatur=off
  Saturation Dynamic1 : simulink/Discontinuities/Saturation Dynamic  OutMin=[]  OutMax=[]  OutDataTypeStr=Inherit: Same as second input  OutDataType=fixdt(1, 16)  OutScaling=2^-10  DoSatur=off
  Subtract1 : Sum  Inputs=+-
  Subtract4 : Sum  Inputs=+-
  Subtract5 : Sum  Inputs=-+-
  Omega : Outport
  "Current " : Outport  Port=2
  wires:
  Inductance1/1 -> Integrator2/1
  Inertia1/1 -> Integrator3/1
  Resistance1/1 -> Subtract5/3
  Damping1/1 -> Subtract4/2
  Subtract5/1 -> Inductance1/1
  Saturation Dynamic1/1 -> Subtract5/2
  Gain4/1 -> Subtract5/1
  Subtract4/1 -> Inertia1/1
  Gain3/1 -> Subtract4/1
  Omega_cmd/1 -> Subtract1/1
  Integrator3/1 -> Subtract1/2, Omega/1, Damping1/1, Gain4/1
  Constant/1 -> Saturation Dynamic/3
  Aval_Current/1 -> Saturation Dynamic/1
  Integrator2/1 -> Saturation Dynamic/2
  Voltage/1 -> Saturation Dynamic1/1
  Constant1/1 -> Saturation Dynamic1/3
  Subtract1/1 -> Saturation Dynamic1/2
  Saturation Dynamic/1 -> Resistance1/1, "Current "/1, Gain3/1

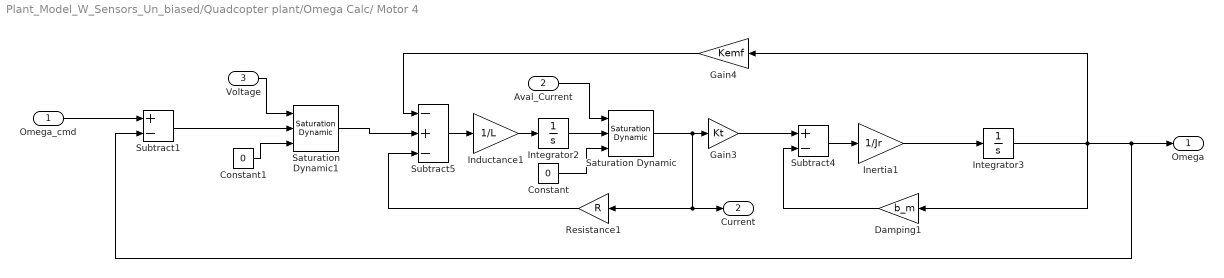
== system Plant_Model_W_Sensors_Un_biased/Quadcopter plant/Omega Calc/ Motor 4 ==
  Omega_cmd : Inport
  Aval_Current : Inport  Port=2
  Voltage : Inport  Port=3
  Constant : Constant  Value=0
  Constant1 : Constant  Value=0
  Damping1 : Gain  Gain=b_m
  Gain3 : Gain  Gain=Kt
  Gain4 : Gain  Gain=Kemf
  Inductance1 : Gain  Gain=1/L
  Inertia1 : Gain  Gain=1/Jr
  Integrator2 : Integrator  LimitOutput=on  LowerSaturationLimit=0
  Integrator3 : Integrator  LimitOutput=on  LowerSaturationLimit=0
  Resistance1 : Gain  Gain=R
  Saturation Dynamic : simulink/Discontinuities/Saturation Dynamic  OutMin=[]  OutMax=[]  OutDataTypeStr=Inherit: Same as second input  OutDataType=fixdt(1, 16)  OutScaling=2^-10  DoSatur=off
  Saturation Dynamic1 : simulink/Discontinuities/Saturation Dynamic  OutMin=[]  OutMax=[]  OutDataTypeStr=Inherit: Same as second input  OutDataType=fixdt(1, 16)  OutScaling=2^-10  DoSatur=off
  Subtract1 : Sum  Inputs=+-
  Subtract4 : Sum  Inputs=+-
  Subtract5 : Sum  Inputs=-+-
  Omega : Outport
  "Current " : Outport  Port=2
  wires:
  Inductance1/1 -> Integrator2/1
  Inertia1/1 -> Integrator3/1
  Resistance1/1 -> Subtract5/3
  Damping1/1 -> Subtract4/2
  Subtract5/1 -> Inductance1/1
  Saturation Dynamic1/1 -> Subtract5/2
  Gain4/1 -> Subtract5/1
  Subtract4/1 -> Inertia1/1
  Gain3/1 -> Subtract4/1
  Omega_cmd/1 -> Subtract1/1
  Integrator3/1 -> Subtract1/2, Omega/1, Damping1/1, Gain4/1
  Constant/1 -> Saturation Dynamic/3
  Aval_Current/1 -> Saturation Dynamic/1
  Integrator2/1 -> Saturation Dynamic/2
  Voltage/1 -> Saturation Dynamic1/1
  Constant1/1 -> Saturation Dynamic1/3
  Subtract1/1 -> Saturation Dynamic1/2
  Saturation Dynamic/1 -> Resistance1/1, "Current "/1, Gain3/1

== matlab function Plant_Model_W_Sensors_Un_biased/IMU/MATLAB Function ==
  data: Xdd input; Ydd input; Zdd input; Phi input; Accel_vec output; Theta input; Psi input
function Accel_vec = World2Body(Xdd,Ydd,Zdd,Phi,Theta,Psi)

Trans_mat=[(cos(Psi)*cos(Theta)), (-sin(Psi)*cos(Phi)+cos(Psi)*sin(Theta)*sin(Phi)), (sin(Psi)*sin(Phi)+cos(Psi)*sin(Theta)*cos(Phi));...
          (sin(Psi)*cos(Theta)), (cos(Psi)*cos(Phi)+sin(Theta)*sin(Psi)*sin(Phi)), (-cos(Psi)*sin(Phi)+sin(Theta)*sin(Psi)*cos(Phi));...
          (-sin(Theta)), (cos(Theta)*sin(Phi)), (cos(Theta)*cos(Phi))];
      
Accel_world=[Xdd;Ydd;Zdd];
Accel_vec=(Trans_mat^-1)*Accel_world;
